simulink model "inverted_pendulum"  (R2021a)
settings: Solver=VariableStepAuto  StartTime=0.0  StopTime=5  FixedStep=0.001  MaxStep=0.0001  RelTol=1e-3
values from neighbouring files (symbols this model uses):
  A = [0          1       0       0 ... (first row only)    [Data.m]
  B = [0 0 0 1/La]'    [Data.m]
  beta = g*(mp*L1 + mw * L2)    (= 0.64746)    [Data.m]    (also in uncertainty.m = g*(mp*L1 + mw * L2))
  bm = 0.018    [Data.m]    (also in uncertainty.m = ureal('bm', 0.018, 'percent', 20))
  bp = 0.038    [Data.m]    (also in uncertainty.m = ureal('bp', 0.038, 'percent', 100))
  C = [1 0 0 0]    [Data.m]
  fs_IMU = 1000    [Data.m]
  g = 9.81    [Data.m]    (also in uncertainty.m)
  ideal_acc_height = 0    [Data.m]
  J1 = Jw + Jp_O    (= 0.0170488)    [Data.m]    (also in uncertainty.m = Jw + Jp_O)
  Jw = J_motor + J_wheel    (= 0.0042488)    [Data.m]    (also in uncertainty.m = J_motor + J_wheel)
  Ke = 1.66e-2    (= 0.0166)    [Data.m]    (also in gear_test.m = gear*Kt; uncertainty.m = ureal('Ke', 1.66e-2, 'percent', 20))
  Ksw = 0.035    [Data.m]    (also in Ksw_test.m = Ksw_v(i))
  Kt = 1    [Data.m]    (also in gear_test.m = gear*0.876; uncertainty.m = ureal('Kt', 1, 'percent', 20))
  L = L_t'    [Data.m]
  La = 3.2e-3    (= 0.0032)    [Data.m]    (also in uncertainty.m = ureal('La', 3.2e-3, 'percent', 20))
  Ra = 40.8    [Data.m]    (also in uncertainty.m = ureal('Ra', 40.8, 'percent', 20))
  real_acc_height = 0.02    [Data.m]
  V_nom = 24    [Data.m]    (also in uncertainty.m)
  wd_IMU = 30000*2*pi    (= 188495.559215)    [Data.m]
  wn = sqrt(mp*g*L2/Jp_O)    [Data.m]
  x0 = [0.3 0 0 0]    [Data.m]
  x0_sw = [pi 0 0 0]    [Data.m]    (also in phase_space.m = [-pi 0 0 0])
undefined symbols (not defined in the file or in its folder): acc_bias, gyro_bias, K
libraries: spsFirstOrderFilterLib x18, simulink x9, dspsigops x2
(part 1 of 2)
settings Model: Creator=jpss8  LastModifiedBy=jpss8

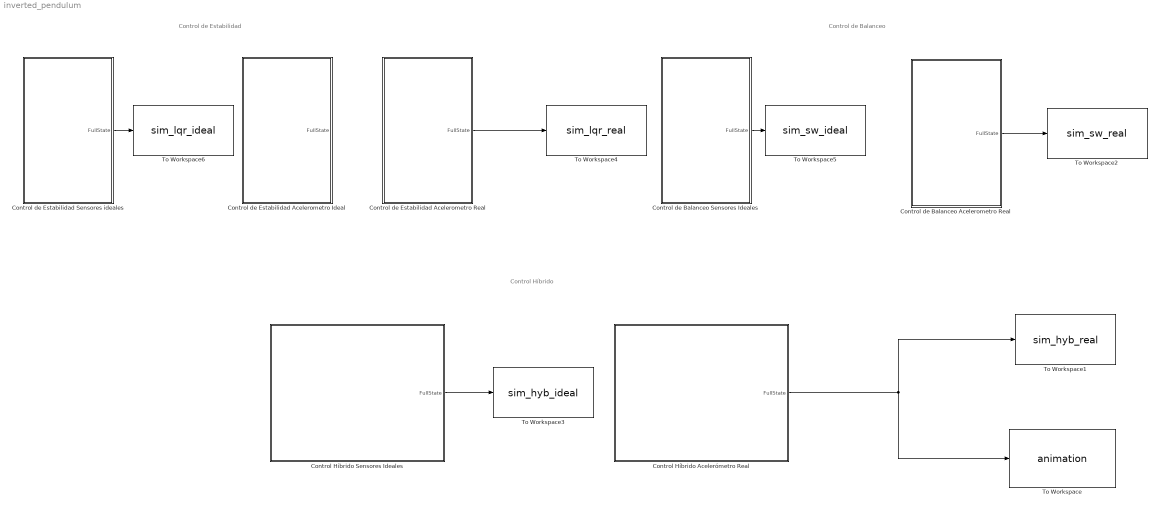
== system inverted_pendulum ==
  note: Control de Estabilidad
  note: Control de Balanceo
  note: Control Híbrido
  Control Híbrido Acelerómetro Real : Subsystem
  Control Híbrido Sensores Ideales : Subsystem
  Control de Balanceo Acelerometro Real : Subsystem
  Control de Balanceo Sensores Ideales : Subsystem
  Control de Estabilidad Acelerometro Ideal : Subsystem
  Control de Estabilidad Acelerometro Real : Subsystem
  Control de Estabilidad Sensores ideales : Subsystem
  To Workspace : ToWorkspace  VariableName=animation  SaveFormat=Structure With Time  SampleTime=-1
  To Workspace1 : ToWorkspace  VariableName=sim_hyb_real  SaveFormat=Structure With Time  SampleTime=-1
  To Workspace2 : ToWorkspace  VariableName=sim_sw_real  SaveFormat=Structure With Time  SampleTime=-1
  To Workspace3 : ToWorkspace  VariableName=sim_hyb_ideal  SaveFormat=Structure With Time  SampleTime=-1
  To Workspace4 : ToWorkspace  VariableName=sim_lqr_real  SaveFormat=Structure With Time  SampleTime=-1
  To Workspace5 : ToWorkspace  VariableName=sim_sw_ideal  SaveFormat=Structure With Time  SampleTime=-1
  To Workspace6 : ToWorkspace  VariableName=sim_lqr_ideal  SaveFormat=Structure With Time  SampleTime=-1
  wires:
  Control Híbrido Acelerómetro Real/1(FullState) -> To Workspace1/1, To Workspace/1
  Control de Estabilidad Sensores ideales/1(FullState) -> To Workspace6/1
  Control de Estabilidad Acelerometro Real/1(FullState) -> To Workspace4/1
  Control de Balanceo Sensores Ideales/1(FullState) -> To Workspace5/1
  Control de Balanceo Acelerometro Real/1(FullState) -> To Workspace2/1
  Control Híbrido Sensores Ideales/1(FullState) -> To Workspace3/1

== system inverted_pendulum/Control Híbrido Acelerómetro Real ==
  note: Saturación Motor DC
  Acondicionamiento de Señal : Subsystem
  Control Híbrido : Subsystem
  Demux : Demux
  Estimación de estados : Subsystem
  Péndulo invertido NL : Subsystem
  Sensores : Subsystem
  Vmax = 24V : Saturate  UpperLimit=V_nom  LowerLimit=-V_nom
  FullState : Outport
  wires:
  Vmax = 24V/1 -> Estimación de estados/1(V), Péndulo invertido NL/1(V)
  Control Híbrido/1(V) -> Vmax = 24V/1
  Demux/1 -> Control Híbrido/1(theta)
  Demux/2 -> Control Híbrido/2(wp)
  Demux/3 -> Control Híbrido/3(wm)
  Demux/4 -> Control Híbrido/4(ia)
  Péndulo invertido NL/1(NL Full State) -> Sensores/1(NL Full State), FullState/1
  Sensores/2(Gyro) -> Acondicionamiento de Señal/1(Gyro)
  Sensores/1(Acc) -> Acondicionamiento de Señal/2(Acc)
  Acondicionamiento de Señal/1(theta_filter) -> Estimación de estados/2(theta)
  Estimación de estados/1(Estado completo estimado) -> Demux/1

== system inverted_pendulum/Control Híbrido Sensores Ideales ==
  note: Saturación Motor DC
  Control Híbrido : Subsystem
  Demux : Demux
  Péndulo invertido NL : Subsystem
  Vmax = 24V : Saturate  UpperLimit=V_nom  LowerLimit=-V_nom
  FullState : Outport
  wires:
  Vmax = 24V/1 -> Péndulo invertido NL/1(V)
  Control Híbrido/1(V) -> Vmax = 24V/1
  Demux/1 -> Control Híbrido/1(theta)
  Demux/2 -> Control Híbrido/2(wp)
  Demux/3 -> Control Híbrido/3(wm)
  Demux/4 -> Control Híbrido/4(ia)
  Péndulo invertido NL/1(NL Full State) -> FullState/1, Demux/1

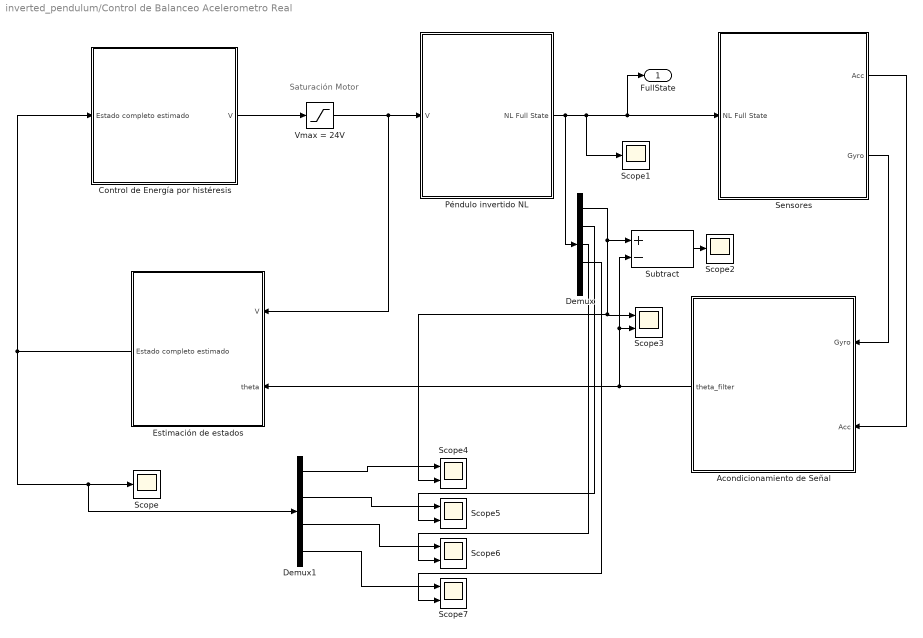
== system inverted_pendulum/Control de Balanceo Acelerometro Real ==
  note: Saturación Motor
  Acondicionamiento de Señal : Subsystem
  Control de Energía por histéresis : Subsystem
  Demux : Demux  Outputs=5
  Demux1 : Demux
  Estimación de estados : Subsystem
  Péndulo invertido NL : Subsystem
  Scope : Scope
  Scope1 : Scope
  Scope2 : Scope
  Scope{3..7} (5 alike) : Scope  NumInputPorts=2
  Sensores : Subsystem
  Subtract : Sum  Inputs=+-
  Vmax = 24V : Saturate  UpperLimit=V_nom  LowerLimit=-V_nom
  FullState : Outport
  wires:
  Vmax = 24V/1 -> Estimación de estados/1(V), Péndulo invertido NL/1(V)
  Control de Energía por histéresis/1(V) -> Vmax = 24V/1
  Péndulo invertido NL/1(NL Full State) -> Demux/1, Scope1/1, FullState/1, Sensores/1(NL Full State)
  Sensores/2(Gyro) -> Acondicionamiento de Señal/1(Gyro)
  Sensores/1(Acc) -> Acondicionamiento de Señal/2(Acc)
  Estimación de estados/1(Estado completo estimado) -> Control de Energía por histéresis/1(Estado completo estimado), Demux1/1, Scope/1
  Demux/1 -> Scope4/2, Scope3/1, Subtract/1
  Subtract/1 -> Scope2/1
  Acondicionamiento de Señal/1(theta_filter) -> Estimación de estados/2(theta), Scope3/2, Subtract/2
  Demux1/1 -> Scope4/1
  Demux1/2 -> Scope5/1
  Demux1/3 -> Scope6/1
  Demux1/4 -> Scope7/1
  Demux/2 -> Scope5/2
  Demux/3 -> Scope6/2
  Demux/4 -> Scope7/2

== system inverted_pendulum/Control de Balanceo Sensores Ideales ==
  note: DC Motor Saturation
  Control de Energía por histéresis : Subsystem
  Gain : Gain
  Péndulo invertido NL : Subsystem
  Vmax = 24V : Saturate  UpperLimit=V_nom  LowerLimit=-V_nom
  FullState : Outport
  wires:
  Vmax = 24V/1 -> Péndulo invertido NL/1(V)
  Control de Energía por histéresis/1(V) -> Vmax = 24V/1
  Gain/1 -> Control de Energía por histéresis/1(Estado completo estimado)
  Péndulo invertido NL/1(NL Full State) -> Gain/1, FullState/1

== system inverted_pendulum/Control de Estabilidad Acelerometro Ideal ==
  note: Saturación Motor DC
  Acondicionamiento de Señal : Subsystem
  Control LQR : Subsystem
  Estimación de estados : Subsystem
  Péndulo invertido NL : Subsystem
  Sensores : Subsystem
  Vmax = 24V : Saturate  UpperLimit=V_nom  LowerLimit=-V_nom
  FullState : Outport
  wires:
  Vmax = 24V/1 -> Péndulo invertido NL/1(V), Estimación de estados/1(V)
  Control LQR/1(V) -> Vmax = 24V/1
  Sensores/1(Acc) -> Acondicionamiento de Señal/1(Acc)
  Acondicionamiento de Señal/1(theta) -> Estimación de estados/2(theta)
  Péndulo invertido NL/1(NL Full State) -> FullState/1, Sensores/1(NL Full State)
  Estimación de estados/1(Estado completo estimado) -> Control LQR/1(Estado estimado)

== system inverted_pendulum/Control de Estabilidad Acelerometro Real ==
  Acondicionamiento de Señal : Subsystem
  Control LQR : Subsystem
  Estimación de estados : Subsystem
  Péndulo invertido NL : Subsystem
  Scope : Scope
  Scope1 : Scope
  Scope2 : Scope
  Sensores : Subsystem
  Vmax = 24V : Saturate  UpperLimit=V_nom  LowerLimit=-V_nom
  FullState : Outport
  wires:
  Vmax = 24V/1 -> Estimación de estados/1(V), Péndulo invertido NL/1(V)
  Control LQR/1(V) -> Vmax = 24V/1
  Sensores/1(Acc) -> Acondicionamiento de Señal/2(Acc)
  Péndulo invertido NL/1(NL Full State) -> Sensores/1(NL Full State), Scope/1, FullState/1
  Sensores/2(Gyro) -> Acondicionamiento de Señal/1(Gyro)
  Acondicionamiento de Señal/1(theta_filter) -> Estimación de estados/2(theta), Scope1/1
  Estimación de estados/1(Estado completo estimado) -> Scope2/1, Control LQR/1(Estado estimado)

== system inverted_pendulum/Control de Estabilidad Sensores ideales ==
  note: Saturación Motor DC
  Control LQR : Subsystem
  Gain : Gain
  Péndulo invertido NL : Subsystem
  Vmax = 24V : Saturate  UpperLimit=V_nom  LowerLimit=-V_nom
  FullState : Outport
  wires:
  Vmax = 24V/1 -> Péndulo invertido NL/1(V)
  Control LQR/1(V) -> Vmax = 24V/1
  Gain/1 -> Control LQR/1(Estado medido)
  Péndulo invertido NL/1(NL Full State) -> Gain/1, FullState/1

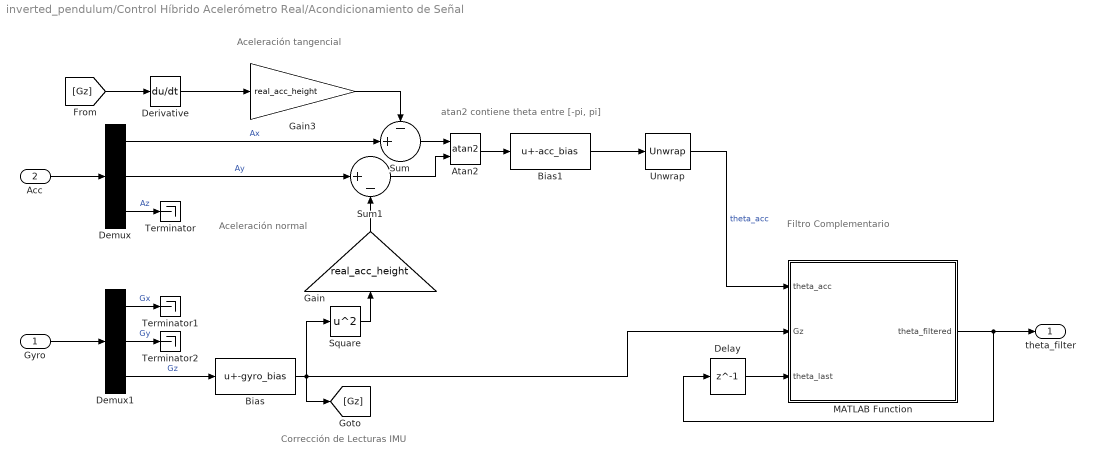
== system inverted_pendulum/Control Híbrido Acelerómetro Real/Acondicionamiento de Señal ==
  note: atan2 contiene theta entre [-pi, pi]
  note: Filtro Complementario
  note: Aceleración tangencial
  note: Aceleración normal
  note: Corrección de Lecturas IMU
  Gyro : Inport
  Acc : Inport  Port=2
  Atan2 : Trigonometry  Operator=atan2
  Bias : Bias  Bias=-gyro_bias
  Bias1 : Bias  Bias=-acc_bias
  Delay : Delay  DelayLength=1  InitialCondition=x0_sw(1)  SampleTime=1/fs_IMU
  Demux : Demux  Outputs=3
  Demux1 : Demux  Outputs=3
  Derivative : Derivative
  Gain : Gain  Gain=real_acc_height
  Gain3 : Gain  Gain=real_acc_height
  MATLAB Function : MATLAB Function  TreatAsAtomicUnit=on
  Square : Math  Operator=square  SaturateOnIntegerOverflow=on
  Sum : Sum  Inputs=-+|
  Sum1 : Sum  Inputs=|+-
  Terminator : Terminator
  Terminator1 : Terminator
  Terminator2 : Terminator
  Unwrap : dspsigops/Unwrap  tol=pi  InputProcessing=Columns as channels (frame based)  running=off
  theta_filter : Outport
  wires:
  Gyro/1 -> Demux1/1
  Acc/1 -> Demux/1
  Demux/1 -> Sum/2  "Ax"
  Demux/3 -> Terminator/1  "Az"
  Sum/1 -> Atan2/1
  Atan2/1 -> Bias1/1
  Demux1/1 -> Terminator1/1  "Gx"
  Demux1/2 -> Terminator2/1  "Gy"
  Demux1/3 -> Bias/1  "Gz"
  MATLAB Function/1(theta_filtered) -> theta_filter/1, Delay/1
  Delay/1 -> MATLAB Function/3(theta_last)
  Unwrap/1 -> MATLAB Function/1(theta_acc)  "theta_acc"
  Demux/2 -> Sum1/1  "Ay"
  Sum1/1 -> Atan2/2
  Bias/1 -> Square/1, [Gz], MATLAB Function/2(Gz)
  Bias1/1 -> Unwrap/1
  Square/1 -> Gain/1
  Gain/1 -> Sum1/2
  Derivative/1 -> Gain3/1
  Gain3/1 -> Sum/1
  [Gz] -> Derivative/1

== system inverted_pendulum/Control Híbrido Acelerómetro Real/Control Híbrido ==
  theta : Inport  OutDataTypeStr=double  PortDimensions=1
  wp : Inport  Port=2  OutDataTypeStr=double  PortDimensions=1
  wm : Inport  Port=3  OutDataTypeStr=double  PortDimensions=1
  ia : Inport  Port=4  OutDataTypeStr=double  PortDimensions=1
  Balanceo : Subsystem
  LQR - Estabilidad : Subsystem
  Lógica de decisión : Subsystem
  Merge : Merge
  V : Outport
  wires:
  Merge/1 -> V/1
  Balanceo/1(V) -> Merge/1
  LQR - Estabilidad/1(V) -> Merge/2
  wp/1 -> Balanceo/2(wp), LQR - Estabilidad/2(wp)  "wp"
  wm/1 -> Balanceo/3(wm), LQR - Estabilidad/3(wm)  "wm"
  ia/1 -> Balanceo/4(ia), LQR - Estabilidad/4(ia)
  theta/1 -> Lógica de decisión/1(theta), Balanceo/1(theta), LQR - Estabilidad/1(theta)
  Lógica de decisión/1(Balanceo) -> Balanceo/Action
  Lógica de decisión/2(Estabilidad) -> LQR - Estabilidad/Action

== system inverted_pendulum/Control Híbrido Acelerómetro Real/Estimación de estados ==
  V : Inport
  theta : Inport  Port=2
  Constant : Constant  Value=A
  Gain : Gain  Gain=L  Multiplication=Matrix(K*u)
  Gain1 : Gain  Gain=C  Multiplication=Matrix(K*u)
  Gain3 : Gain  Gain=B  Multiplication=Matrix(K*u)
  Integrator : Integrator  InitialCondition=x0_sw
  MATLAB Function : MATLAB Function  TreatAsAtomicUnit=on
  Sum : Sum  Inputs=|+-
  Sum1 : Sum  Inputs=+++
  Estado completo estimado : Outport
  wires:
  theta/1 -> Sum/1
  V/1 -> Gain3/1
  Integrator/1 -> Gain1/1, Estado completo estimado/1, MATLAB Function/1(x)
  Gain3/1 -> Sum1/2
  Sum1/1 -> Integrator/1
  MATLAB Function/1(F) -> Sum1/3
  Sum/1 -> Gain/1
  Gain1/1 -> Sum/2
  Gain/1 -> Sum1/1
  Constant/1 -> MATLAB Function/2(A)

== system inverted_pendulum/Control Híbrido Acelerómetro Real/Péndulo invertido NL ==
  V : Inport
  Motor CC + Rueda : Subsystem
  Mux : Mux  Inputs=5
  Péndulo invertido : Subsystem
  NL Full State : Outport
  wires:
  Mux/1 -> NL Full State/1
  Péndulo invertido/2(wp) -> Mux/2  "wp"
  Péndulo invertido/1(theta) -> Mux/1  "theta"
  Motor CC + Rueda/1(wm) -> Mux/3, Péndulo invertido/1(wm)  "wm"
  Motor CC + Rueda/2(ia) -> Péndulo invertido/2(ia), Mux/4  "ia"
  V/1 -> Motor CC + Rueda/1(V)
  Péndulo invertido/3(d2theta) -> Mux/5  "d2theta"

== system inverted_pendulum/Control Híbrido Acelerómetro Real/Sensores ==
  NL Full State : Inport
  Demux : Demux  Outputs=5
  IMU : Subsystem
  Terminator : Terminator
  Terminator1 : Terminator
  Acc : Outport
  Gyro : Outport  Port=2
  wires:
  NL Full State/1 -> Demux/1
  Demux/2 -> IMU/2(wp)
  Demux/1 -> IMU/1(theta)
  Demux/4 -> Terminator/1
  IMU/2(G) -> Gyro/1
  IMU/1(A) -> Acc/1
  Demux/5 -> IMU/3(d2theta)
  Demux/3 -> Terminator1/1

== system inverted_pendulum/Control Híbrido Sensores Ideales/Control Híbrido ==
  theta : Inport  OutDataTypeStr=double  PortDimensions=1
  wp : Inport  Port=2  OutDataTypeStr=double  PortDimensions=1
  wm : Inport  Port=3  OutDataTypeStr=double  PortDimensions=1
  ia : Inport  Port=4  OutDataTypeStr=double  PortDimensions=1
  Balanceo : Subsystem
  LQR - Estabilidad : Subsystem
  Lógica de decisión : Subsystem
  Merge : Merge
  V : Outport
  wires:
  Merge/1 -> V/1
  theta/1 -> Lógica de decisión/1(theta), Balanceo/1(theta), LQR - Estabilidad/1(theta)
  Balanceo/1(V) -> Merge/1
  LQR - Estabilidad/1(V) -> Merge/2
  wp/1 -> Balanceo/2(wp), LQR - Estabilidad/2(wp)  "wp"
  wm/1 -> Balanceo/3(wm), LQR - Estabilidad/3(wm)  "wm"
  ia/1 -> Balanceo/4(ia), LQR - Estabilidad/4(ia)
  Lógica de decisión/1(Balanceo) -> Balanceo/Action
  Lógica de decisión/2(Estabilidad) -> LQR - Estabilidad/Action

== system inverted_pendulum/Control Híbrido Sensores Ideales/Péndulo invertido NL ==
  V : Inport
  Motor CC + Rueda : Subsystem
  Mux : Mux
  Péndulo invertido : Subsystem
  Terminator : Terminator
  NL Full State : Outport
  wires:
  Mux/1 -> NL Full State/1
  Péndulo invertido/2(wp) -> Mux/2  "wp"
  Péndulo invertido/1(theta) -> Mux/1  "theta"
  Motor CC + Rueda/1(wm) -> Mux/3, Péndulo invertido/1(wm)  "wm"
  Motor CC + Rueda/2(ia) -> Péndulo invertido/2(ia), Mux/4  "ia"
  V/1 -> Motor CC + Rueda/1(V)
  Péndulo invertido/3(d2theta) -> Terminator/1  "d2theta"

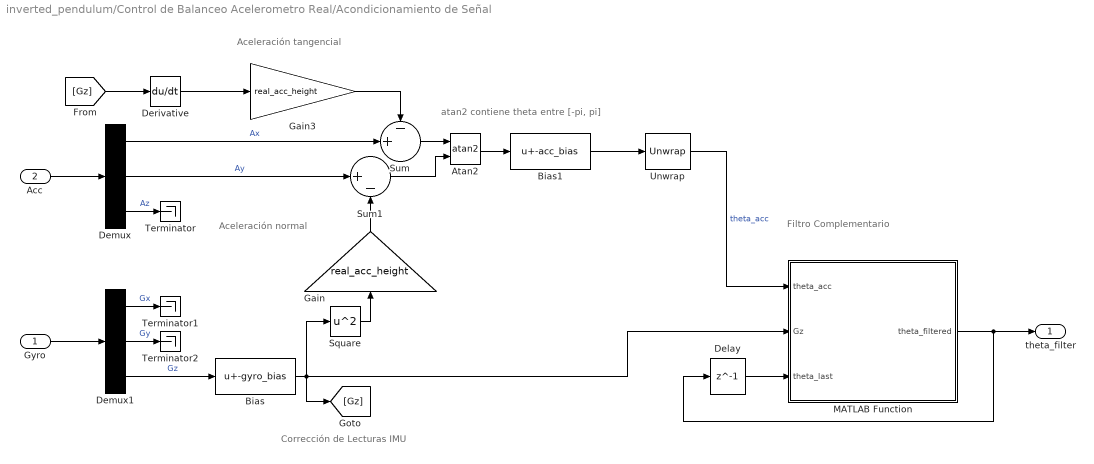
== system inverted_pendulum/Control de Balanceo Acelerometro Real/Acondicionamiento de Señal ==
  note: atan2 contiene theta entre [-pi, pi]
  note: Filtro Complementario
  note: Aceleración tangencial
  note: Aceleración normal
  note: Corrección de Lecturas IMU
  Gyro : Inport
  Acc : Inport  Port=2
  Atan2 : Trigonometry  Operator=atan2
  Bias : Bias  Bias=-gyro_bias
  Bias1 : Bias  Bias=-acc_bias
  Delay : Delay  DelayLength=1  InitialCondition=x0_sw(1)  SampleTime=1/fs_IMU
  Demux : Demux  Outputs=3
  Demux1 : Demux  Outputs=3
  Derivative : Derivative
  Gain : Gain  Gain=real_acc_height
  Gain3 : Gain  Gain=real_acc_height
  MATLAB Function : MATLAB Function  TreatAsAtomicUnit=on
  Square : Math  Operator=square  SaturateOnIntegerOverflow=on
  Sum : Sum  Inputs=-+|
  Sum1 : Sum  Inputs=|+-
  Terminator : Terminator
  Terminator1 : Terminator
  Terminator2 : Terminator
  Unwrap : dspsigops/Unwrap  tol=pi  InputProcessing=Columns as channels (frame based)  running=off
  theta_filter : Outport
  wires:
  Gyro/1 -> Demux1/1
  Acc/1 -> Demux/1
  Demux/1 -> Sum/2  "Ax"
  Demux/3 -> Terminator/1  "Az"
  Sum/1 -> Atan2/1
  Atan2/1 -> Bias1/1
  Demux1/1 -> Terminator1/1  "Gx"
  Demux1/2 -> Terminator2/1  "Gy"
  Demux1/3 -> Bias/1  "Gz"
  MATLAB Function/1(theta_filtered) -> theta_filter/1, Delay/1
  Delay/1 -> MATLAB Function/3(theta_last)
  Unwrap/1 -> MATLAB Function/1(theta_acc)  "theta_acc"
  Demux/2 -> Sum1/1  "Ay"
  Sum1/1 -> Atan2/2
  Bias/1 -> Square/1, [Gz], MATLAB Function/2(Gz)
  Bias1/1 -> Unwrap/1
  Square/1 -> Gain/1
  Gain/1 -> Sum1/2
  Derivative/1 -> Gain3/1
  Gain3/1 -> Sum/1
  [Gz] -> Derivative/1

== system inverted_pendulum/Control de Balanceo Acelerometro Real/Control de Energía por histéresis ==
  Estado completo estimado : Inport
  Cálculo de Energía : Subsystem
  Demux : Demux
  Gain : Gain
  Gain1 : Gain  Gain=Ksw
  Gain2 : Gain  Gain=-V_nom
  Product : Product
  Scope : Scope
  Scope1 : Scope
  Scope2 : Scope
  Sum : Sum  Inputs=|+-
  Terminator : Terminator
  V : Outport
  wires:
  Cálculo de Energía/1(Eref-E) -> Scope1/1, Product/1
  Estado completo estimado/1 -> Demux/1
  Demux/2 -> Product/2, Cálculo de Energía/2(wp)  "wp"
  Product/1 -> Gain/1
  Gain/1 -> Sum/1
  Demux/3 -> Gain1/1  "wm"
  Gain1/1 -> Sum/2
  Sum/1 -> Gain2/1
  Demux/4 -> Terminator/1
  Demux/1 -> Cálculo de Energía/1(theta), Scope/1
  Gain2/1 -> Scope2/1, V/1

== system inverted_pendulum/Control de Balanceo Acelerometro Real/Estimación de estados ==
  V : Inport
  theta : Inport  Port=2
  Constant : Constant  Value=A
  Gain : Gain  Gain=L  Multiplication=Matrix(K*u)
  Gain1 : Gain  Gain=C  Multiplication=Matrix(K*u)
  Gain3 : Gain  Gain=B  Multiplication=Matrix(K*u)
  Integrator : Integrator  InitialCondition=x0_sw
  MATLAB Function : MATLAB Function  TreatAsAtomicUnit=on
  Sum : Sum  Inputs=|+-
  Sum1 : Sum  Inputs=+++
  Estado completo estimado : Outport
  wires:
  theta/1 -> Sum/1
  V/1 -> Gain3/1
  Integrator/1 -> Gain1/1, Estado completo estimado/1, MATLAB Function/1(x)
  Gain3/1 -> Sum1/2
  Sum1/1 -> Integrator/1
  MATLAB Function/1(F) -> Sum1/3
  Sum/1 -> Gain/1
  Gain1/1 -> Sum/2
  Gain/1 -> Sum1/1
  Constant/1 -> MATLAB Function/2(A)

== system inverted_pendulum/Control de Balanceo Acelerometro Real/Péndulo invertido NL ==
  V : Inport
  Motor CC + Rueda : Subsystem
  Mux : Mux  Inputs=5
  Péndulo invertido : Subsystem
  NL Full State : Outport
  wires:
  Mux/1 -> NL Full State/1
  Péndulo invertido/2(wp) -> Mux/2  "wp"
  Péndulo invertido/1(theta) -> Mux/1  "theta"
  Motor CC + Rueda/1(wm) -> Mux/3, Péndulo invertido/1(wm)  "wm"
  Motor CC + Rueda/2(ia) -> Péndulo invertido/2(ia), Mux/4  "ia"
  V/1 -> Motor CC + Rueda/1(V)
  Péndulo invertido/3(d2theta) -> Mux/5  "d2theta"

== system inverted_pendulum/Control de Balanceo Acelerometro Real/Sensores ==
  NL Full State : Inport
  Demux : Demux  Outputs=5
  IMU : Subsystem
  Terminator : Terminator
  Terminator1 : Terminator
  Acc : Outport
  Gyro : Outport  Port=2
  wires:
  NL Full State/1 -> Demux/1
  Demux/2 -> IMU/2(wp)
  Demux/1 -> IMU/1(theta)
  Demux/4 -> Terminator/1
  IMU/2(G) -> Gyro/1
  IMU/1(A) -> Acc/1
  Demux/5 -> IMU/3(d2theta)
  Demux/3 -> Terminator1/1

== system inverted_pendulum/Control de Balanceo Sensores Ideales/Control de Energía por histéresis ==
  Estado completo estimado : Inport
  Cálculo de Energía : Subsystem
  Demux : Demux
  Gain : Gain
  Gain1 : Gain  Gain=Ksw
  Gain2 : Gain  Gain=-V_nom
  Product : Product
  Sum : Sum  Inputs=|+-
  Terminator : Terminator
  V : Outport
  wires:
  Cálculo de Energía/1(Eref-E) -> Product/1
  Estado completo estimado/1 -> Demux/1
  Demux/2 -> Product/2, Cálculo de Energía/2(wp)  "wp"
  Product/1 -> Gain/1
  Gain/1 -> Sum/1
  Demux/3 -> Gain1/1  "wm"
  Gain1/1 -> Sum/2
  Sum/1 -> Gain2/1
  Demux/4 -> Terminator/1
  Demux/1 -> Cálculo de Energía/1(theta)
  Gain2/1 -> V/1

== system inverted_pendulum/Control de Balanceo Sensores Ideales/Péndulo invertido NL ==
  V : Inport
  Motor CC + Rueda : Subsystem
  Mux : Mux
  Péndulo invertido : Subsystem
  Terminator : Terminator
  NL Full State : Outport
  wires:
  Mux/1 -> NL Full State/1
  Péndulo invertido/2(wp) -> Mux/2  "wp"
  Péndulo invertido/1(theta) -> Mux/1  "theta"
  Motor CC + Rueda/1(wm) -> Mux/3, Péndulo invertido/1(wm)  "wm"
  Motor CC + Rueda/2(ia) -> Péndulo invertido/2(ia), Mux/4  "ia"
  V/1 -> Motor CC + Rueda/1(V)
  Péndulo invertido/3(d2theta) -> Terminator/1  "d2theta"

== system inverted_pendulum/Control de Estabilidad Acelerometro Ideal/Acondicionamiento de Señal ==
  Acc : Inport
  Atan2 : Trigonometry  Operator=atan2
  Demux : Demux  Outputs=3
  Terminator : Terminator
  theta : Outport
  wires:
  Acc/1 -> Demux/1
  Demux/1 -> Atan2/1  "Ax"
  Demux/2 -> Atan2/2  "Ay"
  Demux/3 -> Terminator/1  "Az"
  Atan2/1 -> theta/1  "theta_acc"

== system inverted_pendulum/Control de Estabilidad Acelerometro Ideal/Control LQR ==
  Estado estimado : Inport
  Gain : Gain  Gain=-K  Multiplication=Matrix(K*u)
  V : Outport
  wires:
  Estado estimado/1 -> Gain/1
  Gain/1 -> V/1

== system inverted_pendulum/Control de Estabilidad Acelerometro Ideal/Estimación de estados ==
  V : Inport
  theta : Inport  Port=2
  Constant : Constant  Value=A
  Gain : Gain  Gain=L  Multiplication=Matrix(K*u)
  Gain1 : Gain  Gain=C  Multiplication=Matrix(K*u)
  Gain3 : Gain  Gain=B  Multiplication=Matrix(K*u)
  Integrator : Integrator  InitialCondition=x0_sw
  MATLAB Function : MATLAB Function  TreatAsAtomicUnit=on
  Sum : Sum  Inputs=|+-
  Sum1 : Sum  Inputs=+++
  Estado completo estimado : Outport
  wires:
  theta/1 -> Sum/1
  V/1 -> Gain3/1
  Integrator/1 -> Gain1/1, Estado completo estimado/1, MATLAB Function/1(x)
  Gain3/1 -> Sum1/2
  Sum1/1 -> Integrator/1
  MATLAB Function/1(F) -> Sum1/3
  Sum/1 -> Gain/1
  Gain1/1 -> Sum/2
  Gain/1 -> Sum1/1
  Constant/1 -> MATLAB Function/2(A)

== system inverted_pendulum/Control de Estabilidad Acelerometro Ideal/Péndulo invertido NL ==
  V : Inport
  Motor CC + Rueda : Subsystem
  Mux : Mux  Inputs=5
  Péndulo invertido : Subsystem
  NL Full State : Outport
  wires:
  Mux/1 -> NL Full State/1
  Péndulo invertido/2(wp) -> Mux/2  "wp"
  Péndulo invertido/1(theta) -> Mux/1  "theta"
  Motor CC + Rueda/1(wm) -> Mux/3, Péndulo invertido/1(wm)  "wm"
  Motor CC + Rueda/2(ia) -> Péndulo invertido/2(ia), Mux/4  "ia"
  V/1 -> Motor CC + Rueda/1(V)
  Péndulo invertido/3(d2theta) -> Mux/5  "d2theta"

== system inverted_pendulum/Control de Estabilidad Acelerometro Ideal/Sensores ==
  NL Full State : Inport
  Demux : Demux  Outputs=5
  IMU : Subsystem
  Terminator : Terminator
  Terminator1 : Terminator
  Acc : Outport
  Gyro : Outport  Port=2
  wires:
  NL Full State/1 -> Demux/1
  Demux/2 -> IMU/2(wp)
  Demux/1 -> IMU/1(theta)
  Demux/4 -> Terminator/1
  IMU/2(G) -> Gyro/1
  IMU/1(A) -> Acc/1
  Demux/5 -> IMU/3(d2theta)
  Demux/3 -> Terminator1/1

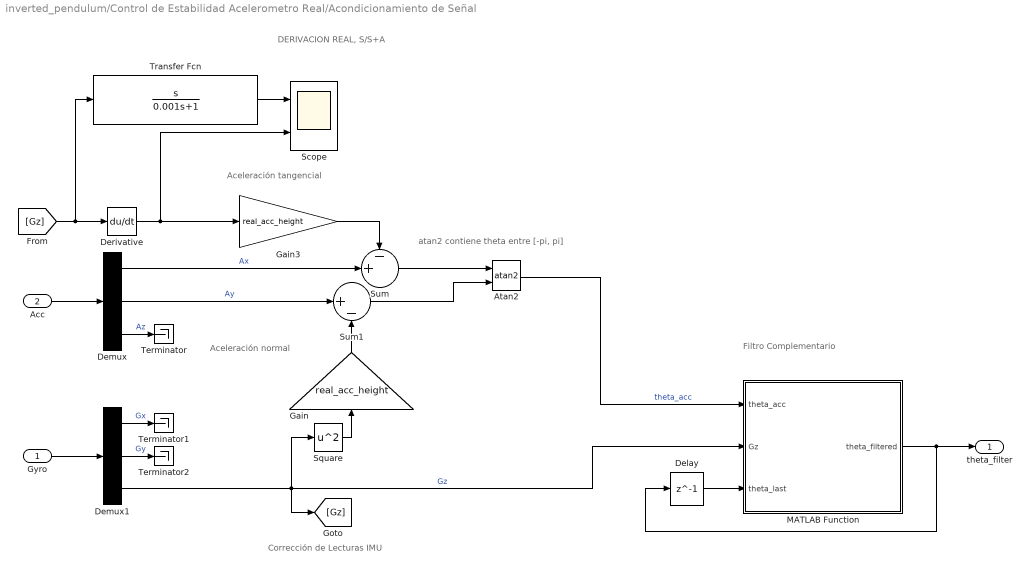
== system inverted_pendulum/Control de Estabilidad Acelerometro Real/Acondicionamiento de Señal ==
  note: DERIVACION REAL, S/S+A
  note: atan2 contiene theta entre [-pi, pi]
  note: Filtro Complementario
  note: Aceleración tangencial
  note: Aceleración normal
  note: Corrección de Lecturas IMU
  Gyro : Inport
  Acc : Inport  Port=2
  Atan2 : Trigonometry  Operator=atan2
  Delay : Delay  DelayLength=1  InitialCondition=x0(1)  SampleTime=1/fs_IMU
  Demux : Demux  Outputs=3
  Demux1 : Demux  Outputs=3
  Derivative : Derivative
  Gain : Gain  Gain=real_acc_height
  Gain3 : Gain  Gain=real_acc_height
  MATLAB Function : MATLAB Function  TreatAsAtomicUnit=on
  Scope : Scope  NumInputPorts=2
  Square : Math  Operator=square  SaturateOnIntegerOverflow=on
  Sum : Sum  Inputs=-+|
  Sum1 : Sum  Inputs=|+-
  Terminator : Terminator
  Terminator1 : Terminator
  Terminator2 : Terminator
  Transfer Fcn : TransferFcn  Numerator=[1 0]  Denominator=[0.001 1]
  theta_filter : Outport
  wires:
  Gyro/1 -> Demux1/1
  Acc/1 -> Demux/1
  Demux/1 -> Sum/2  "Ax"
  Demux/3 -> Terminator/1  "Az"
  Demux1/1 -> Terminator1/1  "Gx"
  Demux1/2 -> Terminator2/1  "Gy"
  Demux1/3 -> Square/1, [Gz], MATLAB Function/2(Gz)  "Gz"
  MATLAB Function/1(theta_filtered) -> theta_filter/1, Delay/1
  Delay/1 -> MATLAB Function/3(theta_last)
  Atan2/1 -> MATLAB Function/1(theta_acc)  "theta_acc"
  Demux/2 -> Sum1/1  "Ay"
  Sum1/1 -> Atan2/2
  Square/1 -> Gain/1
  Gain/1 -> Sum1/2
  Derivative/1 -> Scope/2, Gain3/1
  Gain3/1 -> Sum/1
  [Gz] -> Transfer Fcn/1, Derivative/1
  Sum/1 -> Atan2/1
  Transfer Fcn/1 -> Scope/1

== system inverted_pendulum/Control de Estabilidad Acelerometro Real/Control LQR ==
  Estado estimado : Inport
  Gain : Gain  Gain=-K  Multiplication=Matrix(K*u)
  V : Outport
  wires:
  Estado estimado/1 -> Gain/1
  Gain/1 -> V/1

== system inverted_pendulum/Control de Estabilidad Acelerometro Real/Estimación de estados ==
  V : Inport
  theta : Inport  Port=2
  Constant : Constant  Value=A
  Gain : Gain  Gain=L  Multiplication=Matrix(K*u)
  Gain1 : Gain  Gain=C  Multiplication=Matrix(K*u)
  Gain3 : Gain  Gain=B  Multiplication=Matrix(K*u)
  Integrator : Integrator  InitialCondition=x0_sw
  MATLAB Function : MATLAB Function  TreatAsAtomicUnit=on
  Sum : Sum  Inputs=|+-
  Sum1 : Sum  Inputs=+++
  Estado completo estimado : Outport
  wires:
  theta/1 -> Sum/1
  V/1 -> Gain3/1
  Integrator/1 -> Gain1/1, Estado completo estimado/1, MATLAB Function/1(x)
  Gain3/1 -> Sum1/2
  Sum1/1 -> Integrator/1
  MATLAB Function/1(F) -> Sum1/3
  Sum/1 -> Gain/1
  Gain1/1 -> Sum/2
  Gain/1 -> Sum1/1
  Constant/1 -> MATLAB Function/2(A)

== system inverted_pendulum/Control de Estabilidad Acelerometro Real/Péndulo invertido NL ==
  V : Inport
  Motor CC + Rueda : Subsystem
  Mux : Mux  Inputs=5
  Péndulo invertido : Subsystem
  NL Full State : Outport
  wires:
  Mux/1 -> NL Full State/1
  Péndulo invertido/2(wp) -> Mux/2  "wp"
  Péndulo invertido/1(theta) -> Mux/1  "theta"
  Motor CC + Rueda/1(wm) -> Mux/3, Péndulo invertido/1(wm)  "wm"
  Motor CC + Rueda/2(ia) -> Péndulo invertido/2(ia), Mux/4  "ia"
  V/1 -> Motor CC + Rueda/1(V)
  Péndulo invertido/3(d2theta) -> Mux/5  "d2theta"

== system inverted_pendulum/Control de Estabilidad Acelerometro Real/Sensores ==
  NL Full State : Inport
  Demux : Demux  Outputs=5
  IMU : Subsystem
  Terminator : Terminator
  Terminator1 : Terminator
  Acc : Outport
  Gyro : Outport  Port=2
  wires:
  NL Full State/1 -> Demux/1
  Demux/2 -> IMU/2(wp)
  Demux/1 -> IMU/1(theta)
  Demux/4 -> Terminator/1
  IMU/2(G) -> Gyro/1
  IMU/1(A) -> Acc/1
  Demux/5 -> IMU/3(d2theta)
  Demux/3 -> Terminator1/1

== system inverted_pendulum/Control de Estabilidad Sensores ideales/Control LQR ==
  Estado medido : Inport
  Gain : Gain  Gain=-K  Multiplication=Matrix(K*u)
  V : Outport
  wires:
  Estado medido/1 -> Gain/1
  Gain/1 -> V/1

== system inverted_pendulum/Control de Estabilidad Sensores ideales/Péndulo invertido NL ==
  V : Inport
  Motor CC + Rueda : Subsystem
  Mux : Mux
  Péndulo invertido : Subsystem
  Terminator : Terminator
  NL Full State : Outport
  wires:
  Mux/1 -> NL Full State/1
  Péndulo invertido/2(wp) -> Mux/2  "wp"
  Péndulo invertido/1(theta) -> Mux/1  "theta"
  Motor CC + Rueda/1(wm) -> Mux/3, Péndulo invertido/1(wm)  "wm"
  Motor CC + Rueda/2(ia) -> Péndulo invertido/2(ia), Mux/4  "ia"
  V/1 -> Motor CC + Rueda/1(V)
  Péndulo invertido/3(d2theta) -> Terminator/1

== system inverted_pendulum/Control Híbrido Acelerómetro Real/Control Híbrido/Balanceo ==
  theta : Inport  OutDataTypeStr=double  PortDimensions=1
  wp : Inport  Port=2  OutDataTypeStr=double  PortDimensions=1
  wm : Inport  Port=3  OutDataTypeStr=double  PortDimensions=1
  ia : Inport  Port=4  OutDataTypeStr=double  PortDimensions=1
  Action Port : ActionPort  ActionPortLabel=if(u1 > 0.5 | u1 < -0.5)
  Cálculo de Energía : Subsystem
  Gain : Gain
  Gain1 : Gain  Gain=Ksw
  Gain2 : Gain  Gain=-V_nom
  Product : Product
  Sum : Sum  Inputs=|+-
  Terminator : Terminator
  V : Outport
  wires:
  wp/1 -> Cálculo de Energía/2(wp), Product/2
  theta/1 -> Cálculo de Energía/1(theta)
  Cálculo de Energía/1(Eref-E) -> Product/1
  ia/1 -> Terminator/1
  Gain2/1 -> V/1
  Sum/1 -> Gain2/1
  Gain1/1 -> Sum/2
  Gain/1 -> Sum/1
  Product/1 -> Gain/1
  wm/1 -> Gain1/1

== system inverted_pendulum/Control Híbrido Acelerómetro Real/Control Híbrido/LQR - Estabilidad ==
  theta : Inport
  wp : Inport  Port=2
  wm : Inport  Port=3
  ia : Inport  Port=4
  Action Port : ActionPort  ActionPortLabel=else
  Gain : Gain  Gain=-K  Multiplication=Matrix(K*u)
  Mux : Mux
  V : Outport
  wires:
  Mux/1 -> Gain/1
  theta/1 -> Mux/1
  wp/1 -> Mux/2
  wm/1 -> Mux/3
  ia/1 -> Mux/4
  Gain/1 -> V/1

== system inverted_pendulum/Control Híbrido Acelerómetro Real/Control Híbrido/Lógica de decisión ==
  theta : Inport
  If : If  IfExpression=u1 > 0.5 | u1 < -0.5
  Trigonometric Function : Trigonometry
  Trigonometric Function1 : Trigonometry  Operator=cos
  Trigonometric Function2 : Trigonometry  Operator=atan2
  Balanceo : Outport
  Estabilidad : Outport  Port=2
  wires:
  If/1 -> Balanceo/1
  theta/1 -> Trigonometric Function/1, Trigonometric Function1/1
  If/2 -> Estabilidad/1
  Trigonometric Function1/1 -> Trigonometric Function2/2
  Trigonometric Function2/1 -> If/1
  Trigonometric Function/1 -> Trigonometric Function2/1

== system inverted_pendulum/Control Híbrido Acelerómetro Real/Péndulo invertido NL/Motor CC + Rueda ==
  note: Rueda
  note: Motor CC
  V : Inport
  Gain : Gain  Gain=1/Jw
  Gain1 : Gain  Gain=bm
  Gain2 : Gain  Gain=Kt
  Gain3 : Gain  Gain=1/La
  Gain4 : Gain  Gain=Ra
  Gain5 : Gain  Gain=Ke
  Integrator ia : Integrator  InitialCondition=x0_sw(4)
  Integrator wm : Integrator  InitialCondition=x0_sw(3)
  Sum : Sum  Inputs=|+-
  Sum1 : Sum  Inputs=|+--
  wm : Outport
  ia : Outport  Port=2
  wires:
  Sum/1 -> Gain/1
  Gain/1 -> Integrator wm/1  "d2phi"
  Integrator wm/1 -> wm/1, Gain1/1, Gain5/1  "wm"
  Gain1/1 -> Sum/2
  Gain2/1 -> Sum/1
  Integrator ia/1 -> ia/1, Gain4/1, Gain2/1  "ia"
  Gain3/1 -> Integrator ia/1  "di/dt"
  Sum1/1 -> Gain3/1
  Gain4/1 -> Sum1/3
  V/1 -> Sum1/1  "V"
  Gain5/1 -> Sum1/2

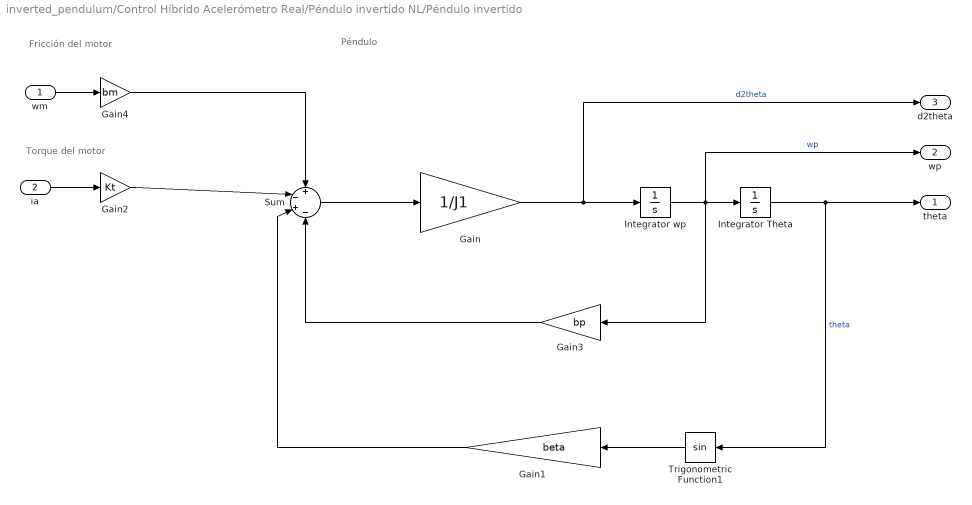
== system inverted_pendulum/Control Híbrido Acelerómetro Real/Péndulo invertido NL/Péndulo invertido ==
  note: Péndulo
  note: Fricción del motor
  note: Torque del motor
  wm : Inport
  ia : Inport  Port=2
  Gain : Gain  Gain=1/J1
  Gain1 : Gain  Gain=beta
  Gain2 : Gain  Gain=Kt
  Gain3 : Gain  Gain=bp
  Gain4 : Gain  Gain=bm
  Integrator Theta : Integrator  InitialCondition=x0_sw(1)  WrappedStateUpperValue=2*pi  WrappedStateLowerValue=0
  Integrator wp : Integrator  InitialCondition=x0_sw(2)
  Sum : Sum  Inputs=+-+-
  Trigonometric Function1 : Trigonometry
  theta : Outport
  wp : Outport  Port=2
  d2theta : Outport  Port=3
  wires:
  Trigonometric Function1/1 -> Gain1/1
  Gain/1 -> d2theta/1, Integrator wp/1  "d2theta"
  Sum/1 -> Gain/1
  Integrator Theta/1 -> Trigonometric Function1/1, theta/1  "theta"
  Integrator wp/1 -> wp/1, Gain3/1, Integrator Theta/1  "wp"
  Gain3/1 -> Sum/4
  Gain1/1 -> Sum/3
  ia/1 -> Gain2/1
  Gain2/1 -> Sum/2
  wm/1 -> Gain4/1
  Gain4/1 -> Sum/1

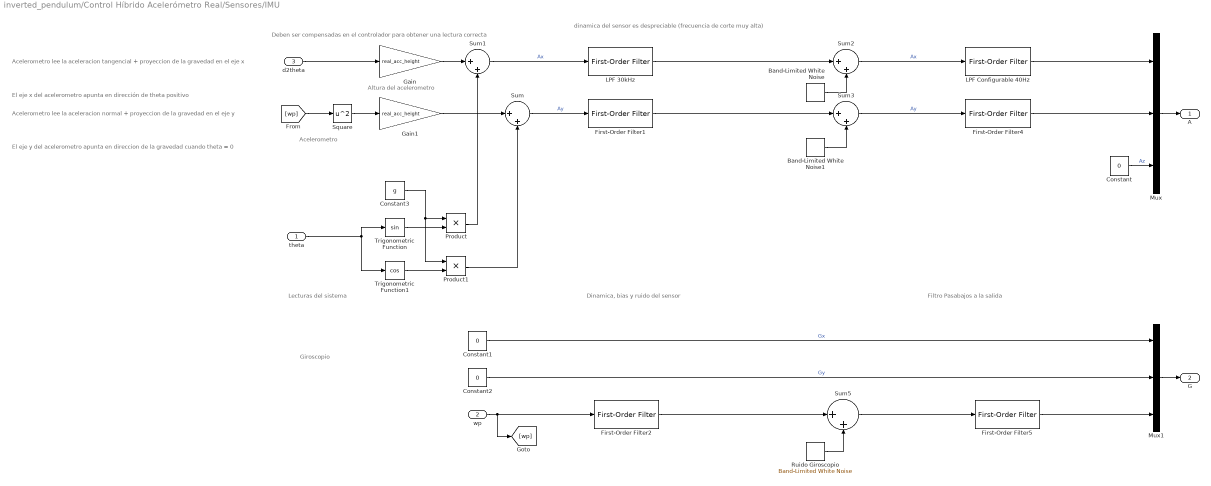
== system inverted_pendulum/Control Híbrido Acelerómetro Real/Sensores/IMU ==
  note: dinamica del sensor es despreciable (frecuencia de corte muy alta)
  note: Dinamica, bias y ruido del sensor
  note: Lecturas del sistema
  note: Acelerometro
  note: Deben ser compensadas en el controlador para obtener una lectura correcta
  note: Acelerometro lee la aceleracion tangencial + proyeccion de la gravedad en el eje x
  note: Altura del acelerometro
  note: El eje y del acelerometro apunta en direccion de la gravedad cuando theta = 0
  note: El eje x del acelerometro apunta en dirección de theta positivo
  note: Acelerometro lee la aceleracion normal + proyeccion de la gravedad en el eje y
  note: Giroscopio
  note: Filtro Pasabajos a la salida
  theta : Inport
  wp : Inport  Port=2
  d2theta : Inport  Port=3
  Band-Limited White Noise : simulink/Sources/Band-Limited White Noise  Cov=acc_noise_power  Ts=1/fs_IMU  seed=[23341]
  Band-Limited White Noise1 : simulink/Sources/Band-Limited White Noise  Cov=acc_noise_power  Ts=1/fs_IMU  seed=[23341]
  Constant : Constant  Value=0
  Constant1 : Constant  Value=0
  Constant2 : Constant  Value=0
  Constant3 : Constant  Value=g
  First-Order Filter{1..2,4..5} (4 alike) : spsFirstOrderFilterLib/First-Order Filter  FilterType=Lowpass  Tc=2*pi/wd_IMU  Ts=0  Initialize=on  Vac_Init=[0, 0, 60]  Vdc_Init=0  PlotResponse=off  FreqRange="[0,  200,  1]"
  Gain : Gain  Gain=real_acc_height
  Gain1 : Gain  Gain=real_acc_height
  LPF 30kHz : spsFirstOrderFilterLib/First-Order Filter  FilterType=Lowpass  Tc=2*pi/wd_IMU  Ts=0  Initialize=on  Vac_Init=[0, 0, 60]  Vdc_Init=0  PlotResponse=off  FreqRange="[0,  200,  1]"
  LPF Configurable 40Hz : spsFirstOrderFilterLib/First-Order Filter  FilterType=Lowpass  Tc=2*pi/wd_IMU  Ts=0  Initialize=on  Vac_Init=[0, 0, 60]  Vdc_Init=0  PlotResponse=off  FreqRange="[0,  200,  1]"
  Mux : Mux  Inputs=3
  Mux1 : Mux  Inputs=3
  Product : Product
  Product1 : Product
  Ruido Giroscopio : simulink/Sources/Band-Limited White Noise  Cov=gyro_noise_power  Ts=1/fs_IMU  seed=[23341]
  Square : Math  Operator=square  SaturateOnIntegerOverflow=on
  Sum{,1..3,5} (5 alike) : Sum  Inputs=|++
  Trigonometric Function : Trigonometry
  Trigonometric Function1 : Trigonometry  Operator=cos
  A : Outport
  G : Outport  Port=2
  wires:
  Constant2/1 -> Mux1/2  "Gy"
  Constant1/1 -> Mux1/1  "Gx"
  Trigonometric Function/1 -> Product/2
  Trigonometric Function1/1 -> Product1/2
  Constant3/1 -> Product1/1, Product/1
  Product1/1 -> Sum/2
  Product/1 -> Sum1/2
  Gain1/1 -> Sum/1
  theta/1 -> Trigonometric Function1/1, Trigonometric Function/1
  Gain/1 -> Sum1/1
  d2theta/1 -> Gain/1
  Square/1 -> Gain1/1
  Constant/1 -> Mux/3  "Az"
  Sum1/1 -> LPF 30kHz/1  "Ax"
  Band-Limited White Noise/1 -> Sum2/2
  Band-Limited White Noise1/1 -> Sum3/2
  Ruido Giroscopio/1 -> Sum5/2
  First-Order Filter1/1 -> Sum3/1
  First-Order Filter2/1 -> Sum5/1
  wp/1 -> First-Order Filter2/1, [wp]
  Mux/1 -> A/1
  Mux1/1 -> G/1
  Sum5/1 -> First-Order Filter5/1
  Sum2/1 -> LPF Configurable 40Hz/1  "Ax"
  Sum3/1 -> First-Order Filter4/1  "Ay"
  [wp] -> Square/1
  Sum/1 -> First-Order Filter1/1  "Ay"
  LPF 30kHz/1 -> Sum2/1
  First-Order Filter4/1 -> Mux/2
  LPF Configurable 40Hz/1 -> Mux/1
  First-Order Filter5/1 -> Mux1/3

== system inverted_pendulum/Control Híbrido Sensores Ideales/Control Híbrido/Balanceo ==
  theta : Inport  OutDataTypeStr=double  PortDimensions=1
  wp : Inport  Port=2  OutDataTypeStr=double  PortDimensions=1
  wm : Inport  Port=3  OutDataTypeStr=double  PortDimensions=1
  ia : Inport  Port=4  OutDataTypeStr=double  PortDimensions=1
  Action Port : ActionPort  ActionPortLabel=if(u1 > 0.5 | u1 < -0.5)
  Cálculo de Energía : Subsystem
  Gain : Gain
  Gain1 : Gain  Gain=Ksw
  Gain2 : Gain  Gain=-V_nom
  Product : Product
  Sum : Sum  Inputs=|+-
  Terminator : Terminator
  V : Outport
  wires:
  wp/1 -> Cálculo de Energía/2(wp), Product/2
  theta/1 -> Cálculo de Energía/1(theta)
  Cálculo de Energía/1(Eref-E) -> Product/1
  ia/1 -> Terminator/1
  Gain2/1 -> V/1
  Sum/1 -> Gain2/1
  Gain1/1 -> Sum/2
  Gain/1 -> Sum/1
  Product/1 -> Gain/1
  wm/1 -> Gain1/1

== system inverted_pendulum/Control Híbrido Sensores Ideales/Control Híbrido/LQR - Estabilidad ==
  theta : Inport
  wp : Inport  Port=2
  wm : Inport  Port=3
  ia : Inport  Port=4
  Action Port : ActionPort  ActionPortLabel=else
  Gain : Gain  Gain=-K  Multiplication=Matrix(K*u)
  Mux : Mux
  V : Outport
  wires:
  Mux/1 -> Gain/1
  theta/1 -> Mux/1
  wp/1 -> Mux/2
  wm/1 -> Mux/3
  ia/1 -> Mux/4
  Gain/1 -> V/1

== system inverted_pendulum/Control Híbrido Sensores Ideales/Control Híbrido/Lógica de decisión ==
  theta : Inport
  If : If  IfExpression=u1 > 0.5 | u1 < -0.5
  Trigonometric Function : Trigonometry
  Trigonometric Function1 : Trigonometry  Operator=cos
  Trigonometric Function2 : Trigonometry  Operator=atan2
  Balanceo : Outport
  Estabilidad : Outport  Port=2
  wires:
  If/1 -> Balanceo/1
  theta/1 -> Trigonometric Function/1, Trigonometric Function1/1
  If/2 -> Estabilidad/1
  Trigonometric Function1/1 -> Trigonometric Function2/2
  Trigonometric Function2/1 -> If/1
  Trigonometric Function/1 -> Trigonometric Function2/1

== system inverted_pendulum/Control Híbrido Sensores Ideales/Péndulo invertido NL/Motor CC + Rueda ==
  note: Rueda
  note: Motor CC
  V : Inport
  Gain : Gain  Gain=1/Jw
  Gain1 : Gain  Gain=bm
  Gain2 : Gain  Gain=Kt
  Gain3 : Gain  Gain=1/La
  Gain4 : Gain  Gain=Ra
  Gain5 : Gain  Gain=Ke
  Integrator ia : Integrator  InitialCondition=x0_sw(4)
  Integrator wm : Integrator  InitialCondition=x0_sw(3)
  Sum : Sum  Inputs=|+-
  Sum1 : Sum  Inputs=|+--
  wm : Outport
  ia : Outport  Port=2
  wires:
  Sum/1 -> Gain/1
  Gain/1 -> Integrator wm/1  "d2phi"
  Integrator wm/1 -> wm/1, Gain1/1, Gain5/1  "wm"
  Gain1/1 -> Sum/2
  Gain2/1 -> Sum/1
  Integrator ia/1 -> ia/1, Gain4/1, Gain2/1  "ia"
  Gain3/1 -> Integrator ia/1  "di/dt"
  Sum1/1 -> Gain3/1
  Gain4/1 -> Sum1/3
  V/1 -> Sum1/1  "V"
  Gain5/1 -> Sum1/2

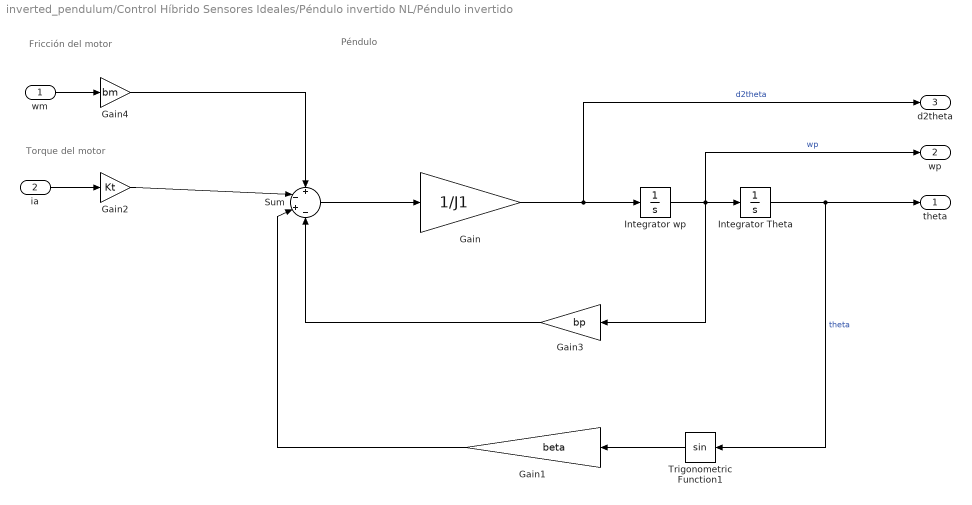
== system inverted_pendulum/Control Híbrido Sensores Ideales/Péndulo invertido NL/Péndulo invertido ==
  note: Péndulo
  note: Fricción del motor
  note: Torque del motor
  wm : Inport
  ia : Inport  Port=2
  Gain : Gain  Gain=1/J1
  Gain1 : Gain  Gain=beta
  Gain2 : Gain  Gain=Kt
  Gain3 : Gain  Gain=bp
  Gain4 : Gain  Gain=bm
  Integrator Theta : Integrator  InitialCondition=x0_sw(1)  WrappedStateUpperValue=2*pi  WrappedStateLowerValue=0
  Integrator wp : Integrator  InitialCondition=x0_sw(2)
  Sum : Sum  Inputs=+-+-
  Trigonometric Function1 : Trigonometry
  theta : Outport
  wp : Outport  Port=2
  d2theta : Outport  Port=3
  wires:
  Trigonometric Function1/1 -> Gain1/1
  Gain/1 -> d2theta/1, Integrator wp/1  "d2theta"
  Sum/1 -> Gain/1
  Integrator Theta/1 -> Trigonometric Function1/1, theta/1  "theta"
  Integrator wp/1 -> wp/1, Gain3/1, Integrator Theta/1  "wp"
  Gain3/1 -> Sum/4
  Gain1/1 -> Sum/3
  ia/1 -> Gain2/1
  Gain2/1 -> Sum/2
  wm/1 -> Gain4/1
  Gain4/1 -> Sum/1

== system inverted_pendulum/Control de Balanceo Acelerometro Real/Control de Energía por histéresis/Cálculo de Energía ==
  note: Energía Potencial
  note: Energía cinética
  note: Energía instantánea
  note: Energía en theta = 0
  theta : Inport
  wp : Inport  Port=2
  Constant : Constant
  Constant1 : Constant  Value=wn^2
  Constant2 : Constant  Value=2
  Divide : Product  Inputs=*/
  Gain : Gain  Gain=1/2
  Square : Math  Operator=square  SaturateOnIntegerOverflow=on
  Sum : Sum  Inputs=|+-
  Sum1 : Sum  Inputs=+++
  Trigonometric Function : Trigonometry  Operator=cos
  Eref-E : Outport
  wires:
  Sum/1 -> Eref-E/1
  Constant2/1 -> Sum/1  "Eref"
  Sum1/1 -> Sum/2  "E"
  Constant/1 -> Sum1/3
  Trigonometric Function/1 -> Sum1/2
  theta/1 -> Trigonometric Function/1  "theta"
  Divide/1 -> Square/1
  wp/1 -> Divide/1  "wp"
  Constant1/1 -> Divide/2  "wn"
  Square/1 -> Gain/1
  Gain/1 -> Sum1/1

== system inverted_pendulum/Control de Balanceo Acelerometro Real/Péndulo invertido NL/Motor CC + Rueda ==
  note: Rueda
  note: Motor CC
  V : Inport
  Gain : Gain  Gain=1/Jw
  Gain1 : Gain  Gain=bm
  Gain2 : Gain  Gain=Kt
  Gain3 : Gain  Gain=1/La
  Gain4 : Gain  Gain=Ra
  Gain5 : Gain  Gain=Ke
  Integrator ia : Integrator  InitialCondition=x0_sw(4)
  Integrator wm : Integrator  InitialCondition=x0_sw(3)
  Sum : Sum  Inputs=|+-
  Sum1 : Sum  Inputs=|+--
  wm : Outport
  ia : Outport  Port=2
  wires:
  Sum/1 -> Gain/1
  Gain/1 -> Integrator wm/1  "d2phi"
  Integrator wm/1 -> wm/1, Gain1/1, Gain5/1  "wm"
  Gain1/1 -> Sum/2
  Gain2/1 -> Sum/1
  Integrator ia/1 -> ia/1, Gain4/1, Gain2/1  "ia"
  Gain3/1 -> Integrator ia/1  "di/dt"
  Sum1/1 -> Gain3/1
  Gain4/1 -> Sum1/3
  V/1 -> Sum1/1  "V"
  Gain5/1 -> Sum1/2

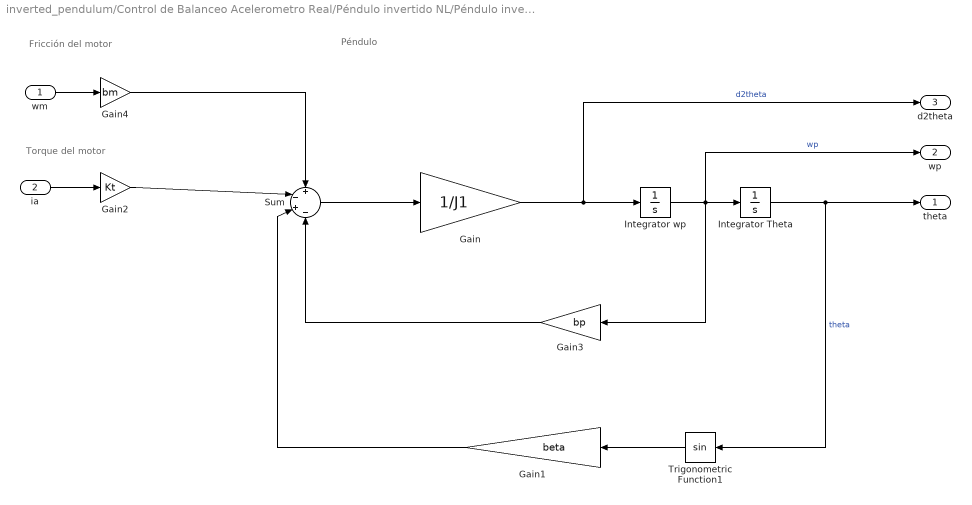
== system inverted_pendulum/Control de Balanceo Acelerometro Real/Péndulo invertido NL/Péndulo invertido ==
  note: Péndulo
  note: Fricción del motor
  note: Torque del motor
  wm : Inport
  ia : Inport  Port=2
  Gain : Gain  Gain=1/J1
  Gain1 : Gain  Gain=beta
  Gain2 : Gain  Gain=Kt
  Gain3 : Gain  Gain=bp
  Gain4 : Gain  Gain=bm
  Integrator Theta : Integrator  InitialCondition=x0_sw(1)  WrappedStateUpperValue=2*pi  WrappedStateLowerValue=0
  Integrator wp : Integrator  InitialCondition=x0_sw(2)
  Sum : Sum  Inputs=+-+-
  Trigonometric Function1 : Trigonometry
  theta : Outport
  wp : Outport  Port=2
  d2theta : Outport  Port=3
  wires:
  Trigonometric Function1/1 -> Gain1/1
  Gain/1 -> d2theta/1, Integrator wp/1  "d2theta"
  Sum/1 -> Gain/1
  Integrator Theta/1 -> Trigonometric Function1/1, theta/1  "theta"
  Integrator wp/1 -> wp/1, Gain3/1, Integrator Theta/1  "wp"
  Gain3/1 -> Sum/4
  Gain1/1 -> Sum/3
  ia/1 -> Gain2/1
  Gain2/1 -> Sum/2
  wm/1 -> Gain4/1
  Gain4/1 -> Sum/1

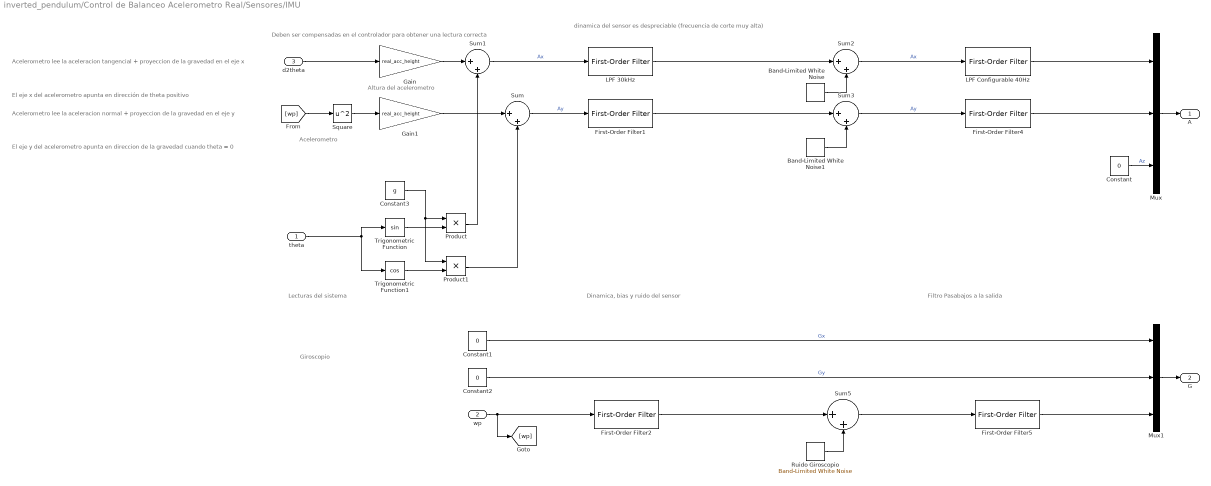
== system inverted_pendulum/Control de Balanceo Acelerometro Real/Sensores/IMU ==
  note: dinamica del sensor es despreciable (frecuencia de corte muy alta)
  note: Dinamica, bias y ruido del sensor
  note: Lecturas del sistema
  note: Acelerometro
  note: Deben ser compensadas en el controlador para obtener una lectura correcta
  note: Acelerometro lee la aceleracion tangencial + proyeccion de la gravedad en el eje x
  note: Altura del acelerometro
  note: El eje y del acelerometro apunta en direccion de la gravedad cuando theta = 0
  note: El eje x del acelerometro apunta en dirección de theta positivo
  note: Acelerometro lee la aceleracion normal + proyeccion de la gravedad en el eje y
  note: Giroscopio
  note: Filtro Pasabajos a la salida
  theta : Inport
  wp : Inport  Port=2
  d2theta : Inport  Port=3
  Band-Limited White Noise : simulink/Sources/Band-Limited White Noise  Cov=acc_noise_power  Ts=1/fs_IMU  seed=[23341]
  Band-Limited White Noise1 : simulink/Sources/Band-Limited White Noise  Cov=acc_noise_power  Ts=1/fs_IMU  seed=[23341]
  Constant : Constant  Value=0
  Constant1 : Constant  Value=0
  Constant2 : Constant  Value=0
  Constant3 : Constant  Value=g
  First-Order Filter{1..2,4..5} (4 alike) : spsFirstOrderFilterLib/First-Order Filter  FilterType=Lowpass  Tc=2*pi/wd_IMU  Ts=0  Initialize=on  Vac_Init=[0, 0, 60]  Vdc_Init=0  PlotResponse=off  FreqRange="[0,  200,  1]"
  Gain : Gain  Gain=real_acc_height
  Gain1 : Gain  Gain=real_acc_height
  LPF 30kHz : spsFirstOrderFilterLib/First-Order Filter  FilterType=Lowpass  Tc=2*pi/wd_IMU  Ts=0  Initialize=on  Vac_Init=[0, 0, 60]  Vdc_Init=0  PlotResponse=off  FreqRange="[0,  200,  1]"
  LPF Configurable 40Hz : spsFirstOrderFilterLib/First-Order Filter  FilterType=Lowpass  Tc=2*pi/wd_IMU  Ts=0  Initialize=on  Vac_Init=[0, 0, 60]  Vdc_Init=0  PlotResponse=off  FreqRange="[0,  200,  1]"
  Mux : Mux  Inputs=3
  Mux1 : Mux  Inputs=3
  Product : Product
  Product1 : Product
  Ruido Giroscopio : simulink/Sources/Band-Limited White Noise  Cov=gyro_noise_power  Ts=1/fs_IMU  seed=[23341]
  Square : Math  Operator=square  SaturateOnIntegerOverflow=on
  Sum{,1..3,5} (5 alike) : Sum  Inputs=|++
  Trigonometric Function : Trigonometry
  Trigonometric Function1 : Trigonometry  Operator=cos
  A : Outport
  G : Outport  Port=2
  wires:
  Constant2/1 -> Mux1/2  "Gy"
  Constant1/1 -> Mux1/1  "Gx"
  Trigonometric Function/1 -> Product/2
  Trigonometric Function1/1 -> Product1/2
  Constant3/1 -> Product1/1, Product/1
  Product1/1 -> Sum/2
  Product/1 -> Sum1/2
  Gain1/1 -> Sum/1
  theta/1 -> Trigonometric Function1/1, Trigonometric Function/1
  Gain/1 -> Sum1/1
  d2theta/1 -> Gain/1
  Square/1 -> Gain1/1
  Constant/1 -> Mux/3  "Az"
  Sum1/1 -> LPF 30kHz/1  "Ax"
  Band-Limited White Noise/1 -> Sum2/2
  Band-Limited White Noise1/1 -> Sum3/2
  Ruido Giroscopio/1 -> Sum5/2
  First-Order Filter1/1 -> Sum3/1
  First-Order Filter2/1 -> Sum5/1
  wp/1 -> First-Order Filter2/1, [wp]
  Mux/1 -> A/1
  Mux1/1 -> G/1
  Sum5/1 -> First-Order Filter5/1
  Sum2/1 -> LPF Configurable 40Hz/1  "Ax"
  Sum3/1 -> First-Order Filter4/1  "Ay"
  [wp] -> Square/1
  Sum/1 -> First-Order Filter1/1  "Ay"
  LPF 30kHz/1 -> Sum2/1
  First-Order Filter4/1 -> Mux/2
  LPF Configurable 40Hz/1 -> Mux/1
  First-Order Filter5/1 -> Mux1/3

== system inverted_pendulum/Control de Balanceo Sensores Ideales/Control de Energía por histéresis/Cálculo de Energía ==
  note: Energía Potencial
  note: Energía cinética
  note: Energía instantánea
  note: Energía en theta = 0
  theta : Inport
  wp : Inport  Port=2
  Constant : Constant
  Constant1 : Constant  Value=wn^2
  Constant2 : Constant  Value=2
  Divide : Product  Inputs=*/
  Gain : Gain  Gain=1/2
  Square : Math  Operator=square  SaturateOnIntegerOverflow=on
  Sum : Sum  Inputs=|+-
  Sum1 : Sum  Inputs=+++
  Trigonometric Function : Trigonometry  Operator=cos
  Eref-E : Outport
  wires:
  Sum/1 -> Eref-E/1
  Constant2/1 -> Sum/1  "Eref"
  Sum1/1 -> Sum/2  "E"
  Constant/1 -> Sum1/3
  Trigonometric Function/1 -> Sum1/2
  theta/1 -> Trigonometric Function/1  "theta"
  Divide/1 -> Square/1
  wp/1 -> Divide/1  "wp"
  Constant1/1 -> Divide/2  "wn"
  Square/1 -> Gain/1
  Gain/1 -> Sum1/1

== system inverted_pendulum/Control de Balanceo Sensores Ideales/Péndulo invertido NL/Motor CC + Rueda ==
  note: Rueda
  note: Motor CC
  V : Inport
  Gain : Gain  Gain=1/Jw
  Gain1 : Gain  Gain=bm
  Gain2 : Gain  Gain=Kt
  Gain3 : Gain  Gain=1/La
  Gain4 : Gain  Gain=Ra
  Gain5 : Gain  Gain=Ke
  Integrator ia : Integrator  InitialCondition=x0_sw(4)
  Integrator wm : Integrator  InitialCondition=x0_sw(3)
  Sum : Sum  Inputs=|+-
  Sum1 : Sum  Inputs=|+--
  wm : Outport
  ia : Outport  Port=2
  wires:
  Sum/1 -> Gain/1
  Gain/1 -> Integrator wm/1  "d2phi"
  Integrator wm/1 -> wm/1, Gain1/1, Gain5/1  "wm"
  Gain1/1 -> Sum/2
  Gain2/1 -> Sum/1
  Integrator ia/1 -> ia/1, Gain4/1, Gain2/1  "ia"
  Gain3/1 -> Integrator ia/1  "di/dt"
  Sum1/1 -> Gain3/1
  Gain4/1 -> Sum1/3
  V/1 -> Sum1/1  "V"
  Gain5/1 -> Sum1/2

== system inverted_pendulum/Control de Balanceo Sensores Ideales/Péndulo invertido NL/Péndulo invertido ==
  note: Péndulo
  note: Fricción del motor
  note: Torque del motor
  wm : Inport
  ia : Inport  Port=2
  Gain : Gain  Gain=1/J1
  Gain1 : Gain  Gain=beta
  Gain2 : Gain  Gain=Kt
  Gain3 : Gain  Gain=bp
  Gain4 : Gain  Gain=bm
  Integrator Theta : Integrator  InitialCondition=x0_sw(1)  WrappedStateUpperValue=2*pi  WrappedStateLowerValue=0
  Integrator wp : Integrator  InitialCondition=x0_sw(2)
  Sum : Sum  Inputs=+-+-
  Trigonometric Function1 : Trigonometry
  theta : Outport
  wp : Outport  Port=2
  d2theta : Outport  Port=3
  wires:
  Trigonometric Function1/1 -> Gain1/1
  Gain/1 -> d2theta/1, Integrator wp/1  "d2theta"
  Sum/1 -> Gain/1
  Integrator Theta/1 -> Trigonometric Function1/1, theta/1  "theta"
  Integrator wp/1 -> wp/1, Gain3/1, Integrator Theta/1  "wp"
  Gain3/1 -> Sum/4
  Gain1/1 -> Sum/3
  ia/1 -> Gain2/1
  Gain2/1 -> Sum/2
  wm/1 -> Gain4/1
  Gain4/1 -> Sum/1

== system inverted_pendulum/Control de Estabilidad Acelerometro Ideal/Péndulo invertido NL/Motor CC + Rueda ==
  note: Rueda
  note: Motor CC
  V : Inport
  Gain : Gain  Gain=1/Jw
  Gain1 : Gain  Gain=bm
  Gain2 : Gain  Gain=Kt
  Gain3 : Gain  Gain=1/La
  Gain4 : Gain  Gain=Ra
  Gain5 : Gain  Gain=Ke
  Integrator ia : Integrator  InitialCondition=x0(4)
  Integrator wm : Integrator  InitialCondition=x0(3)
  Sum : Sum  Inputs=|+-
  Sum1 : Sum  Inputs=|+--
  wm : Outport
  ia : Outport  Port=2
  wires:
  Sum/1 -> Gain/1
  Gain/1 -> Integrator wm/1  "d2phi"
  Integrator wm/1 -> wm/1, Gain1/1, Gain5/1  "wm"
  Gain1/1 -> Sum/2
  Gain2/1 -> Sum/1
  Integrator ia/1 -> ia/1, Gain4/1, Gain2/1  "ia"
  Gain3/1 -> Integrator ia/1  "di/dt"
  Sum1/1 -> Gain3/1
  Gain4/1 -> Sum1/3
  V/1 -> Sum1/1  "V"
  Gain5/1 -> Sum1/2

== system inverted_pendulum/Control de Estabilidad Acelerometro Ideal/Péndulo invertido NL/Péndulo invertido ==
  note: RUIDO DE TORQUE MOTOR POR VARIACION DE LA INDUCTANCIA
  note: VARIACION DEL BRAZO DE TORQUE POR LA TRASLACION HORIZONTAL
  note: COMO MODELAR EL JUEGO
  note: Péndulo
  note: Fricción del motor
  note: Torque del motor
  wm : Inport
  ia : Inport  Port=2
  Gain : Gain  Gain=1/J1
  Gain1 : Gain  Gain=beta
  Gain2 : Gain  Gain=Kt
  Gain3 : Gain  Gain=bp
  Gain4 : Gain  Gain=bm
  Integrator Theta : Integrator  InitialCondition=x0(1)  WrappedStateUpperValue=2*pi  WrappedStateLowerValue=0
  Integrator wp : Integrator  InitialCondition=x0(2)
  Sum : Sum  Inputs=+-+-
  Trigonometric Function1 : Trigonometry
  theta : Outport
  wp : Outport  Port=2
  d2theta : Outport  Port=3
  wires:
  Trigonometric Function1/1 -> Gain1/1
  Gain/1 -> d2theta/1, Integrator wp/1  "d2theta"
  Sum/1 -> Gain/1
  Integrator Theta/1 -> Trigonometric Function1/1, theta/1  "theta"
  Integrator wp/1 -> wp/1, Gain3/1, Integrator Theta/1  "wp"
  Gain3/1 -> Sum/4
  Gain1/1 -> Sum/3
  ia/1 -> Gain2/1
  Gain2/1 -> Sum/2
  wm/1 -> Gain4/1
  Gain4/1 -> Sum/1
